simulink model "sl_drivepoint"  (Simulink 8.3)
settings: Solver=ode3  SolverMode=SingleTasking  StartTime=0.0  StopTime=15.0  RelTol=1e-3
undefined symbols (not defined in the file): xg
libraries: roblocks x1, simulink x1
settings Model: Creator=pic  LastModifiedBy=Administrator  SimulationMode=external
settings DataIOCC: LimitDataPoints=off  ReturnWorkspaceOutputs=on
settings OptimizationCC: ExpressionDepthLimit=2147483647
settings DebuggingCC: SolverPrmCheckMsg=none  FcnCallInpInsideContextMsg=UseLocalSettings
settings HardwareCC: ProdIntDivRoundTo=Zero  ProdEndianess=LittleEndian  ProdHWDeviceType=Generic->32-bit x86 compatible  TargetLongLongMode=on  TargetIntDivRoundTo=Zero  TargetEndianess=LittleEndian  TargetHWDeviceType=MATLAB Host  ProdEqTarget=off
settings RTWCC: SystemTargetFile=rtwin.tlc  GenCodeOnly=on  TemplateMakefile=rtwin.tmf  Description=Real-Time Windows Target  GenerateReport=on  ProcessScript=rtwin_make_rtw_hook  LaunchReport=on  RTWCompilerOptimization=On
settings CodeAppCC: MaxIdLength=95
settings RTWinTargetCC: TargetLibSuffix=_rtwin.lib  TargetPreCompLibLocation=C:\Program Files\MATLAB\R2014a\toolbox\rtw\targets\rtwin\lib\win64

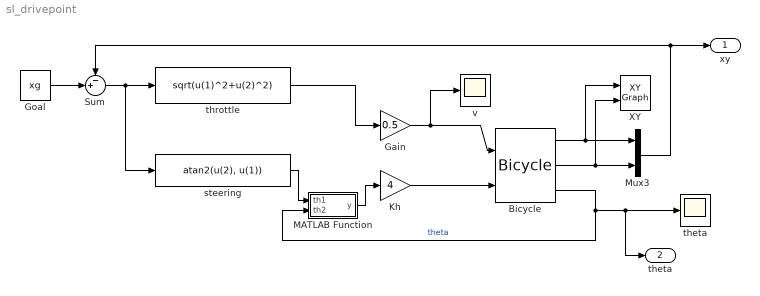
== system sl_drivepoint ==
  Bicycle : roblocks/Dynamics/Bicycle  accel=1  vlim=1  alim=1  L=1  x0=x0  handbrake=0
  Gain : Gain  Gain=0.5
  Goal : Constant  Value=xg
  Kh : Gain  Gain=4
  MATLAB Function : MATLAB Function  TreatAsAtomicUnit=on
  Mux3 : Mux  Inputs=2
  Sum : Sum  Inputs=-+|
  XY : simulink/Sinks/XY Graph  xmin=0  xmax=10  ymin=0  ymax=10  st=-1
  steering : Fcn  Expr=atan2(u(2), u(1))
  theta : Scope
  throttle : Fcn  Expr=sqrt(u(1)^2+u(2)^2)
  v : Scope
      settings: TimeRange=15
  xy : Outport
  "theta " : Outport  Port=2
  wires:
  Bicycle/1 -> Mux3/1, XY/1
  Bicycle/2 -> Mux3/2, XY/2
  Mux3/1 -> xy/1, Sum/1
  Sum/1 -> throttle/1, steering/1
  throttle/1 -> Gain/1
  steering/1 -> MATLAB Function/1(th1)
  Bicycle/3 -> MATLAB Function/2(th2), theta/1, "theta "/1  "theta"
  MATLAB Function/1(y) -> Kh/1
  Gain/1 -> Bicycle/1, v/1
  Goal/1 -> Sum/2
  Kh/1 -> Bicycle/2

== matlab function MATLAB Function ==
  data: th1 input double; y output double; th2 input double
function y = fcn(th1,th2)
%#codegen
if nargin < 2
% THIS IS A BAD IDEA, WHERE IS IT USED?
%         if length(th1) > 1
%             d = th1(1) - th1(2);
%         else
%             d = th1;
%         end
        d = th1;
    else
        d = th1 - th2;
    end

    
    y = mod(d+pi, 2*pi) - pi;
